simulink model "Exercise2"  (Simulink 6.1)
settings: Solver=ode45  StartTime=0.0  StopTime=10.0  RelTol=1e-3
libraries: simulink x1
settings Model: LastModifiedBy=Inderjot
settings DebuggingCC: SolverPrmCheckMsg=warning

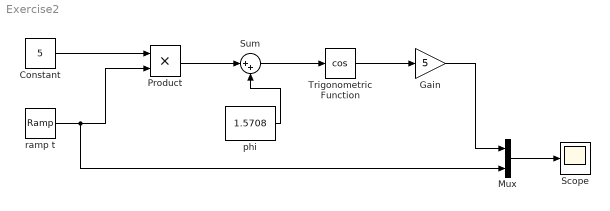
== system Exercise2 ==
  Constant : Constant  Value=5
  Gain : Gain  Gain=5
  Mux : Mux  Inputs=2
  Product : Product  RndMeth=Zero
  Scope : Scope
  Sum : Sum  Inputs=|++
  Trigonometric Function : Trigonometry  Operator=cos
  phi : Constant  Value=1.5708
  ramp t : simulink/Sources/Ramp  slope=1  start=0  X0=0
  wires:
  Constant/1 -> Product/1
  ramp t/1 -> Product/2, Mux/2
  Product/1 -> Sum/1
  Sum/1 -> Trigonometric Function/1
  Trigonometric Function/1 -> Gain/1
  Mux/1 -> Scope/1
  phi/1 -> Sum/2
  Gain/1 -> Mux/1
